simulink model "F16A_Functional"  (R2026a)
settings: Solver=VariableStepAuto
settings Model: DataDictionary=F16A_Functional.sldd  Creator=darsh  LastModifiedBy=darsh

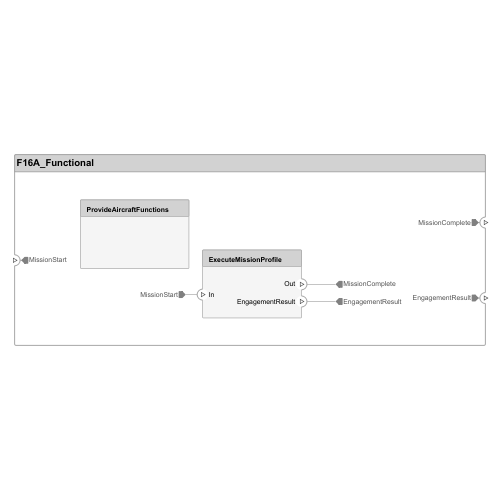
[thumbnail: Simulink's stored preview of the top-level diagram]
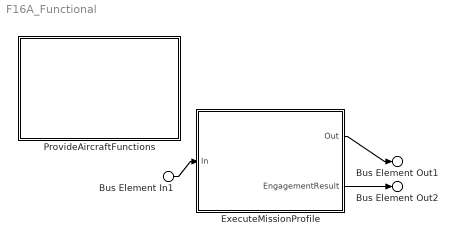
== system F16A_Functional ==
  Bus Element In1 : Inport  PortName=MissionStart
  ExecuteMissionProfile : Subsystem
      settings: PortSchema="{\"entries\":[{\"content\":{\"headerSize\":26,\"margin\":15,\"minimumSpacing\":25,\"sides\":[{\"content\":{\"connectorIds\":[\"In1\"]},\"type\":\"ConnectorPlacement.EquallySpacedRectSide\",\"uuid\":\"f04a52ad-3ae6-4f8c-8d50-829f63627cc8\"},{\"content\":{\"connectorIds\":[\"Out1\",\"Out2\"],\"side\":\"RIGHT\"},\"type\":\"ConnectorPlacement.EquallySpacedRectSide\",\"uuid\":\"fc20b249-404d-406d-9cda-c81cb5f250ae\"},{\"content\":{\"side\":\"TOP\"},\"type\":\"ConnectorPlacement.EquallySpacedRectSide\",\"uuid\":\"dd297750-bae3-47af-9b2d-3c1d29dbfad4\"}]},\"type\":\"ConnectorPlacement.EquallySpacedConnector\",\"uuid\":\"5b4d9ea6-6d9d-4f32-b1f7-36452750b0c8\"}],\"packageUris\":[\"http://schema.mathworks.com/mf0/Connector/R2020b\"],\"version\":\"1.0\"}"
  ProvideAircraftFunctions : Subsystem
      settings: PortSchema="{\"entries\":[{\"content\":{\"headerSize\":26,\"margin\":15,\"minimumSpacing\":25,\"sides\":[{\"content\":{},\"type\":\"ConnectorPlacement.EquallySpacedRectSide\",\"uuid\":\"f04a52ad-3ae6-4f8c-8d50-829f63627cc8\"},{\"content\":{\"side\":\"RIGHT\"},\"type\":\"ConnectorPlacement.EquallySpacedRectSide\",\"uuid\":\"fc20b249-404d-406d-9cda-c81cb5f250ae\"},{\"content\":{\"side\":\"TOP\"},\"type\":\"ConnectorPlacement.EquallySpacedRectSide\",\"uuid\":\"dd297750-bae3-47af-9b2d-3c1d29dbfad4\"}]},\"type\":\"ConnectorPlacement.EquallySpacedConnector\",\"uuid\":\"5b4d9ea6-6d9d-4f32-b1f7-36452750b0c8\"}],\"packageUris\":[\"http://schema.mathworks.com/mf0/Connector/R2020b\"],\"version\":\"1.0\"}"
  Bus Element Out1 : Outport  PortName=MissionComplete
  Bus Element Out2 : Outport  Port=2  PortName=EngagementResult
  wires:
  Bus Element In1/1 -> ExecuteMissionProfile/1(In)
  ExecuteMissionProfile/1(Out) -> Bus Element Out1/1
  ExecuteMissionProfile/2(EngagementResult) -> Bus Element Out2/1

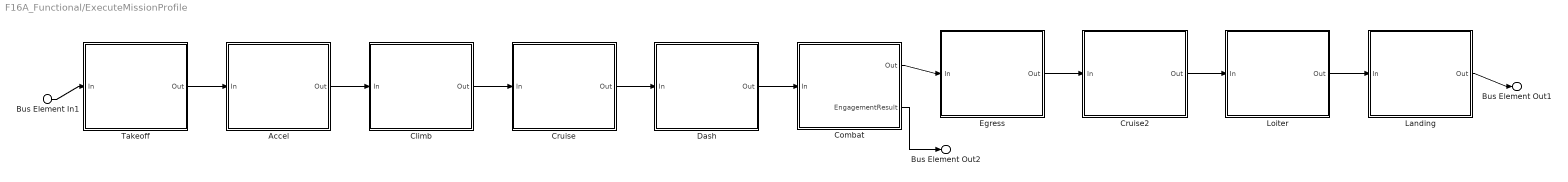
== system F16A_Functional/ExecuteMissionProfile ==
  Bus Element In1 : Inport  PortName=In
  Accel : Subsystem
      settings: PortSchema="{\"entries\":[{\"content\":{\"headerSize\":26,\"margin\":15,\"minimumSpacing\":25,\"sides\":[{\"content\":{\"connectorIds\":[\"In1\"]},\"type\":\"ConnectorPlacement.EquallySpacedRectSide\",\"uuid\":\"f04a52ad-3ae6-4f8c-8d50-829f63627cc8\"},{\"content\":{\"connectorIds\":[\"Out1\"],\"side\":\"RIGHT\"},\"type\":\"ConnectorPlacement.EquallySpacedRectSide\",\"uuid\":\"fc20b249-404d-406d-9cda-c81cb5f250ae\"},{\"content\":{\"side\":\"TOP\"},\"type\":\"ConnectorPlacement.EquallySpacedRectSide\",\"uuid\":\"dd297750-bae3-47af-9b2d-3c1d29dbfad4\"}]},\"type\":\"ConnectorPlacement.EquallySpacedConnector\",\"uuid\":\"5b4d9ea6-6d9d-4f32-b1f7-36452750b0c8\"}],\"packageUris\":[\"http://schema.mathworks.com/mf0/Connector/R2020b\"],\"version\":\"1.0\"}"
  Climb : Subsystem
      settings: PortSchema="{\"entries\":[{\"content\":{\"headerSize\":26,\"margin\":15,\"minimumSpacing\":25,\"sides\":[{\"content\":{\"connectorIds\":[\"In1\"]},\"type\":\"ConnectorPlacement.EquallySpacedRectSide\",\"uuid\":\"f04a52ad-3ae6-4f8c-8d50-829f63627cc8\"},{\"content\":{\"connectorIds\":[\"Out1\"],\"side\":\"RIGHT\"},\"type\":\"ConnectorPlacement.EquallySpacedRectSide\",\"uuid\":\"fc20b249-404d-406d-9cda-c81cb5f250ae\"},{\"content\":{\"side\":\"TOP\"},\"type\":\"ConnectorPlacement.EquallySpacedRectSide\",\"uuid\":\"dd297750-bae3-47af-9b2d-3c1d29dbfad4\"}]},\"type\":\"ConnectorPlacement.EquallySpacedConnector\",\"uuid\":\"5b4d9ea6-6d9d-4f32-b1f7-36452750b0c8\"}],\"packageUris\":[\"http://schema.mathworks.com/mf0/Connector/R2020b\"],\"version\":\"1.0\"}"
  Combat : Subsystem
      settings: PortSchema="{\"entries\":[{\"content\":{\"headerSize\":26,\"margin\":15,\"minimumSpacing\":25,\"sides\":[{\"content\":{\"connectorIds\":[\"In1\"]},\"type\":\"ConnectorPlacement.EquallySpacedRectSide\",\"uuid\":\"f04a52ad-3ae6-4f8c-8d50-829f63627cc8\"},{\"content\":{\"connectorIds\":[\"Out1\",\"Out2\"],\"side\":\"RIGHT\"},\"type\":\"ConnectorPlacement.EquallySpacedRectSide\",\"uuid\":\"fc20b249-404d-406d-9cda-c81cb5f250ae\"},{\"content\":{\"side\":\"TOP\"},\"type\":\"ConnectorPlacement.EquallySpacedRectSide\",\"uuid\":\"dd297750-bae3-47af-9b2d-3c1d29dbfad4\"}]},\"type\":\"ConnectorPlacement.EquallySpacedConnector\",\"uuid\":\"5b4d9ea6-6d9d-4f32-b1f7-36452750b0c8\"}],\"packageUris\":[\"http://schema.mathworks.com/mf0/Connector/R2020b\"],\"version\":\"1.0\"}"
  Cruise : Subsystem
      settings: PortSchema="{\"entries\":[{\"content\":{\"headerSize\":26,\"margin\":15,\"minimumSpacing\":25,\"sides\":[{\"content\":{\"connectorIds\":[\"In1\"]},\"type\":\"ConnectorPlacement.EquallySpacedRectSide\",\"uuid\":\"f04a52ad-3ae6-4f8c-8d50-829f63627cc8\"},{\"content\":{\"connectorIds\":[\"Out1\"],\"side\":\"RIGHT\"},\"type\":\"ConnectorPlacement.EquallySpacedRectSide\",\"uuid\":\"fc20b249-404d-406d-9cda-c81cb5f250ae\"},{\"content\":{\"side\":\"TOP\"},\"type\":\"ConnectorPlacement.EquallySpacedRectSide\",\"uuid\":\"dd297750-bae3-47af-9b2d-3c1d29dbfad4\"}]},\"type\":\"ConnectorPlacement.EquallySpacedConnector\",\"uuid\":\"5b4d9ea6-6d9d-4f32-b1f7-36452750b0c8\"}],\"packageUris\":[\"http://schema.mathworks.com/mf0/Connector/R2020b\"],\"version\":\"1.0\"}"
  Cruise2 : Subsystem
      settings: PortSchema="{\"entries\":[{\"content\":{\"headerSize\":26,\"margin\":15,\"minimumSpacing\":25,\"sides\":[{\"content\":{\"connectorIds\":[\"In1\"]},\"type\":\"ConnectorPlacement.EquallySpacedRectSide\",\"uuid\":\"f04a52ad-3ae6-4f8c-8d50-829f63627cc8\"},{\"content\":{\"connectorIds\":[\"Out1\"],\"side\":\"RIGHT\"},\"type\":\"ConnectorPlacement.EquallySpacedRectSide\",\"uuid\":\"fc20b249-404d-406d-9cda-c81cb5f250ae\"},{\"content\":{\"side\":\"TOP\"},\"type\":\"ConnectorPlacement.EquallySpacedRectSide\",\"uuid\":\"dd297750-bae3-47af-9b2d-3c1d29dbfad4\"}]},\"type\":\"ConnectorPlacement.EquallySpacedConnector\",\"uuid\":\"5b4d9ea6-6d9d-4f32-b1f7-36452750b0c8\"}],\"packageUris\":[\"http://schema.mathworks.com/mf0/Connector/R2020b\"],\"version\":\"1.0\"}"
  Dash : Subsystem
      settings: PortSchema="{\"entries\":[{\"content\":{\"headerSize\":26,\"margin\":15,\"minimumSpacing\":25,\"sides\":[{\"content\":{\"connectorIds\":[\"In1\"]},\"type\":\"ConnectorPlacement.EquallySpacedRectSide\",\"uuid\":\"f04a52ad-3ae6-4f8c-8d50-829f63627cc8\"},{\"content\":{\"connectorIds\":[\"Out1\"],\"side\":\"RIGHT\"},\"type\":\"ConnectorPlacement.EquallySpacedRectSide\",\"uuid\":\"fc20b249-404d-406d-9cda-c81cb5f250ae\"},{\"content\":{\"side\":\"TOP\"},\"type\":\"ConnectorPlacement.EquallySpacedRectSide\",\"uuid\":\"dd297750-bae3-47af-9b2d-3c1d29dbfad4\"}]},\"type\":\"ConnectorPlacement.EquallySpacedConnector\",\"uuid\":\"5b4d9ea6-6d9d-4f32-b1f7-36452750b0c8\"}],\"packageUris\":[\"http://schema.mathworks.com/mf0/Connector/R2020b\"],\"version\":\"1.0\"}"
  Egress : Subsystem
      settings: PortSchema="{\"entries\":[{\"content\":{\"headerSize\":26,\"margin\":15,\"minimumSpacing\":25,\"sides\":[{\"content\":{\"connectorIds\":[\"In1\"]},\"type\":\"ConnectorPlacement.EquallySpacedRectSide\",\"uuid\":\"f04a52ad-3ae6-4f8c-8d50-829f63627cc8\"},{\"content\":{\"connectorIds\":[\"Out1\"],\"side\":\"RIGHT\"},\"type\":\"ConnectorPlacement.EquallySpacedRectSide\",\"uuid\":\"fc20b249-404d-406d-9cda-c81cb5f250ae\"},{\"content\":{\"side\":\"TOP\"},\"type\":\"ConnectorPlacement.EquallySpacedRectSide\",\"uuid\":\"dd297750-bae3-47af-9b2d-3c1d29dbfad4\"}]},\"type\":\"ConnectorPlacement.EquallySpacedConnector\",\"uuid\":\"5b4d9ea6-6d9d-4f32-b1f7-36452750b0c8\"}],\"packageUris\":[\"http://schema.mathworks.com/mf0/Connector/R2020b\"],\"version\":\"1.0\"}"
  Landing : Subsystem
      settings: PortSchema="{\"entries\":[{\"content\":{\"headerSize\":26,\"margin\":15,\"minimumSpacing\":25,\"sides\":[{\"content\":{\"connectorIds\":[\"In1\"]},\"type\":\"ConnectorPlacement.EquallySpacedRectSide\",\"uuid\":\"f04a52ad-3ae6-4f8c-8d50-829f63627cc8\"},{\"content\":{\"connectorIds\":[\"Out1\"],\"side\":\"RIGHT\"},\"type\":\"ConnectorPlacement.EquallySpacedRectSide\",\"uuid\":\"fc20b249-404d-406d-9cda-c81cb5f250ae\"},{\"content\":{\"side\":\"TOP\"},\"type\":\"ConnectorPlacement.EquallySpacedRectSide\",\"uuid\":\"dd297750-bae3-47af-9b2d-3c1d29dbfad4\"}]},\"type\":\"ConnectorPlacement.EquallySpacedConnector\",\"uuid\":\"5b4d9ea6-6d9d-4f32-b1f7-36452750b0c8\"}],\"packageUris\":[\"http://schema.mathworks.com/mf0/Connector/R2020b\"],\"version\":\"1.0\"}"
  Loiter : Subsystem
      settings: PortSchema="{\"entries\":[{\"content\":{\"headerSize\":26,\"margin\":15,\"minimumSpacing\":25,\"sides\":[{\"content\":{\"connectorIds\":[\"In1\"]},\"type\":\"ConnectorPlacement.EquallySpacedRectSide\",\"uuid\":\"f04a52ad-3ae6-4f8c-8d50-829f63627cc8\"},{\"content\":{\"connectorIds\":[\"Out1\"],\"side\":\"RIGHT\"},\"type\":\"ConnectorPlacement.EquallySpacedRectSide\",\"uuid\":\"fc20b249-404d-406d-9cda-c81cb5f250ae\"},{\"content\":{\"side\":\"TOP\"},\"type\":\"ConnectorPlacement.EquallySpacedRectSide\",\"uuid\":\"dd297750-bae3-47af-9b2d-3c1d29dbfad4\"}]},\"type\":\"ConnectorPlacement.EquallySpacedConnector\",\"uuid\":\"5b4d9ea6-6d9d-4f32-b1f7-36452750b0c8\"}],\"packageUris\":[\"http://schema.mathworks.com/mf0/Connector/R2020b\"],\"version\":\"1.0\"}"
  Takeoff : Subsystem
      settings: PortSchema="{\"entries\":[{\"content\":{\"headerSize\":26,\"margin\":15,\"minimumSpacing\":25,\"sides\":[{\"content\":{\"connectorIds\":[\"In1\"]},\"type\":\"ConnectorPlacement.EquallySpacedRectSide\",\"uuid\":\"f04a52ad-3ae6-4f8c-8d50-829f63627cc8\"},{\"content\":{\"connectorIds\":[\"Out1\"],\"side\":\"RIGHT\"},\"type\":\"ConnectorPlacement.EquallySpacedRectSide\",\"uuid\":\"fc20b249-404d-406d-9cda-c81cb5f250ae\"},{\"content\":{\"side\":\"TOP\"},\"type\":\"ConnectorPlacement.EquallySpacedRectSide\",\"uuid\":\"dd297750-bae3-47af-9b2d-3c1d29dbfad4\"}]},\"type\":\"ConnectorPlacement.EquallySpacedConnector\",\"uuid\":\"5b4d9ea6-6d9d-4f32-b1f7-36452750b0c8\"}],\"packageUris\":[\"http://schema.mathworks.com/mf0/Connector/R2020b\"],\"version\":\"1.0\"}"
  Bus Element Out1 : Outport  PortName=Out
  Bus Element Out2 : Outport  Port=2  PortName=EngagementResult
  wires:
  Bus Element In1/1 -> Takeoff/1(In)
  Takeoff/1(Out) -> Accel/1(In)
  Accel/1(Out) -> Climb/1(In)
  Climb/1(Out) -> Cruise/1(In)
  Cruise/1(Out) -> Dash/1(In)
  Combat/2(EngagementResult) -> Bus Element Out2/1
  Dash/1(Out) -> Combat/1(In)
  Combat/1(Out) -> Egress/1(In)
  Cruise2/1(Out) -> Loiter/1(In)
  Egress/1(Out) -> Cruise2/1(In)
  Landing/1(Out) -> Bus Element Out1/1
  Loiter/1(Out) -> Landing/1(In)

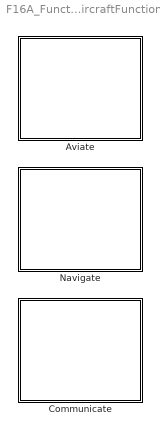
== system F16A_Functional/ProvideAircraftFunctions ==
  Aviate : Subsystem
      settings: PortSchema="{\"entries\":[{\"content\":{\"headerSize\":26,\"margin\":15,\"minimumSpacing\":25,\"sides\":[{\"content\":{},\"type\":\"ConnectorPlacement.EquallySpacedRectSide\",\"uuid\":\"f04a52ad-3ae6-4f8c-8d50-829f63627cc8\"},{\"content\":{\"side\":\"RIGHT\"},\"type\":\"ConnectorPlacement.EquallySpacedRectSide\",\"uuid\":\"fc20b249-404d-406d-9cda-c81cb5f250ae\"},{\"content\":{\"side\":\"TOP\"},\"type\":\"ConnectorPlacement.EquallySpacedRectSide\",\"uuid\":\"dd297750-bae3-47af-9b2d-3c1d29dbfad4\"}]},\"type\":\"ConnectorPlacement.EquallySpacedConnector\",\"uuid\":\"5b4d9ea6-6d9d-4f32-b1f7-36452750b0c8\"}],\"packageUris\":[\"http://schema.mathworks.com/mf0/Connector/R2020b\"],\"version\":\"1.0\"}"
  Communicate : Subsystem
      settings: PortSchema="{\"entries\":[{\"content\":{\"headerSize\":26,\"margin\":15,\"minimumSpacing\":25,\"sides\":[{\"content\":{},\"type\":\"ConnectorPlacement.EquallySpacedRectSide\",\"uuid\":\"f04a52ad-3ae6-4f8c-8d50-829f63627cc8\"},{\"content\":{\"side\":\"RIGHT\"},\"type\":\"ConnectorPlacement.EquallySpacedRectSide\",\"uuid\":\"fc20b249-404d-406d-9cda-c81cb5f250ae\"},{\"content\":{\"side\":\"TOP\"},\"type\":\"ConnectorPlacement.EquallySpacedRectSide\",\"uuid\":\"dd297750-bae3-47af-9b2d-3c1d29dbfad4\"}]},\"type\":\"ConnectorPlacement.EquallySpacedConnector\",\"uuid\":\"5b4d9ea6-6d9d-4f32-b1f7-36452750b0c8\"}],\"packageUris\":[\"http://schema.mathworks.com/mf0/Connector/R2020b\"],\"version\":\"1.0\"}"
  Navigate : Subsystem
      settings: PortSchema="{\"entries\":[{\"content\":{\"headerSize\":26,\"margin\":15,\"minimumSpacing\":25,\"sides\":[{\"content\":{},\"type\":\"ConnectorPlacement.EquallySpacedRectSide\",\"uuid\":\"f04a52ad-3ae6-4f8c-8d50-829f63627cc8\"},{\"content\":{\"side\":\"RIGHT\"},\"type\":\"ConnectorPlacement.EquallySpacedRectSide\",\"uuid\":\"fc20b249-404d-406d-9cda-c81cb5f250ae\"},{\"content\":{\"side\":\"TOP\"},\"type\":\"ConnectorPlacement.EquallySpacedRectSide\",\"uuid\":\"dd297750-bae3-47af-9b2d-3c1d29dbfad4\"}]},\"type\":\"ConnectorPlacement.EquallySpacedConnector\",\"uuid\":\"5b4d9ea6-6d9d-4f32-b1f7-36452750b0c8\"}],\"packageUris\":[\"http://schema.mathworks.com/mf0/Connector/R2020b\"],\"version\":\"1.0\"}"

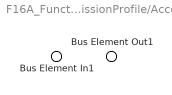
== system F16A_Functional/ExecuteMissionProfile/Accel ==
  Bus Element In1 : Inport  PortName=In
  Bus Element Out1 : Outport  PortName=Out

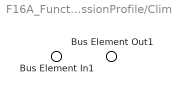
== system F16A_Functional/ExecuteMissionProfile/Climb ==
  Bus Element In1 : Inport  PortName=In
  Bus Element Out1 : Outport  PortName=Out

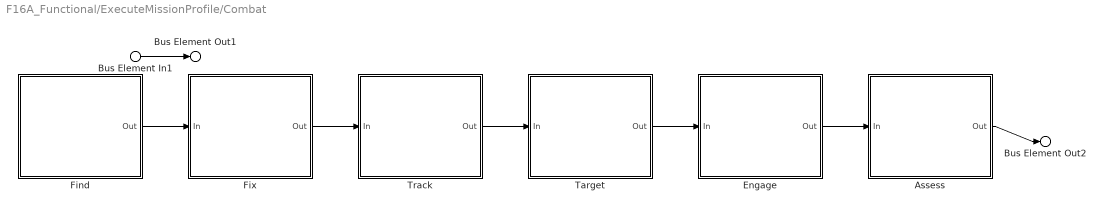
== system F16A_Functional/ExecuteMissionProfile/Combat ==
  Bus Element In1 : Inport  PortName=In
  Assess : Subsystem
      settings: PortSchema="{\"entries\":[{\"content\":{\"headerSize\":26,\"margin\":15,\"minimumSpacing\":25,\"sides\":[{\"content\":{\"connectorIds\":[\"In1\"]},\"type\":\"ConnectorPlacement.EquallySpacedRectSide\",\"uuid\":\"f04a52ad-3ae6-4f8c-8d50-829f63627cc8\"},{\"content\":{\"connectorIds\":[\"Out1\"],\"side\":\"RIGHT\"},\"type\":\"ConnectorPlacement.EquallySpacedRectSide\",\"uuid\":\"fc20b249-404d-406d-9cda-c81cb5f250ae\"},{\"content\":{\"side\":\"TOP\"},\"type\":\"ConnectorPlacement.EquallySpacedRectSide\",\"uuid\":\"dd297750-bae3-47af-9b2d-3c1d29dbfad4\"}]},\"type\":\"ConnectorPlacement.EquallySpacedConnector\",\"uuid\":\"5b4d9ea6-6d9d-4f32-b1f7-36452750b0c8\"}],\"packageUris\":[\"http://schema.mathworks.com/mf0/Connector/R2020b\"],\"version\":\"1.0\"}"
  Engage : Subsystem
      settings: PortSchema="{\"entries\":[{\"content\":{\"headerSize\":26,\"margin\":15,\"minimumSpacing\":25,\"sides\":[{\"content\":{\"connectorIds\":[\"In1\"]},\"type\":\"ConnectorPlacement.EquallySpacedRectSide\",\"uuid\":\"f04a52ad-3ae6-4f8c-8d50-829f63627cc8\"},{\"content\":{\"connectorIds\":[\"Out1\"],\"side\":\"RIGHT\"},\"type\":\"ConnectorPlacement.EquallySpacedRectSide\",\"uuid\":\"fc20b249-404d-406d-9cda-c81cb5f250ae\"},{\"content\":{\"side\":\"TOP\"},\"type\":\"ConnectorPlacement.EquallySpacedRectSide\",\"uuid\":\"dd297750-bae3-47af-9b2d-3c1d29dbfad4\"}]},\"type\":\"ConnectorPlacement.EquallySpacedConnector\",\"uuid\":\"5b4d9ea6-6d9d-4f32-b1f7-36452750b0c8\"}],\"packageUris\":[\"http://schema.mathworks.com/mf0/Connector/R2020b\"],\"version\":\"1.0\"}"
  Find : Subsystem
      settings: PortSchema="{\"entries\":[{\"content\":{\"headerSize\":26,\"margin\":15,\"minimumSpacing\":25,\"sides\":[{\"content\":{},\"type\":\"ConnectorPlacement.EquallySpacedRectSide\",\"uuid\":\"f04a52ad-3ae6-4f8c-8d50-829f63627cc8\"},{\"content\":{\"connectorIds\":[\"Out1\"],\"side\":\"RIGHT\"},\"type\":\"ConnectorPlacement.EquallySpacedRectSide\",\"uuid\":\"fc20b249-404d-406d-9cda-c81cb5f250ae\"},{\"content\":{\"side\":\"TOP\"},\"type\":\"ConnectorPlacement.EquallySpacedRectSide\",\"uuid\":\"dd297750-bae3-47af-9b2d-3c1d29dbfad4\"}]},\"type\":\"ConnectorPlacement.EquallySpacedConnector\",\"uuid\":\"5b4d9ea6-6d9d-4f32-b1f7-36452750b0c8\"}],\"packageUris\":[\"http://schema.mathworks.com/mf0/Connector/R2020b\"],\"version\":\"1.0\"}"
  Fix : Subsystem
      settings: PortSchema="{\"entries\":[{\"content\":{\"headerSize\":26,\"margin\":15,\"minimumSpacing\":25,\"sides\":[{\"content\":{\"connectorIds\":[\"In1\"]},\"type\":\"ConnectorPlacement.EquallySpacedRectSide\",\"uuid\":\"f04a52ad-3ae6-4f8c-8d50-829f63627cc8\"},{\"content\":{\"connectorIds\":[\"Out1\"],\"side\":\"RIGHT\"},\"type\":\"ConnectorPlacement.EquallySpacedRectSide\",\"uuid\":\"fc20b249-404d-406d-9cda-c81cb5f250ae\"},{\"content\":{\"side\":\"TOP\"},\"type\":\"ConnectorPlacement.EquallySpacedRectSide\",\"uuid\":\"dd297750-bae3-47af-9b2d-3c1d29dbfad4\"}]},\"type\":\"ConnectorPlacement.EquallySpacedConnector\",\"uuid\":\"5b4d9ea6-6d9d-4f32-b1f7-36452750b0c8\"}],\"packageUris\":[\"http://schema.mathworks.com/mf0/Connector/R2020b\"],\"version\":\"1.0\"}"
  Target : Subsystem
      settings: PortSchema="{\"entries\":[{\"content\":{\"headerSize\":26,\"margin\":15,\"minimumSpacing\":25,\"sides\":[{\"content\":{\"connectorIds\":[\"In1\"]},\"type\":\"ConnectorPlacement.EquallySpacedRectSide\",\"uuid\":\"f04a52ad-3ae6-4f8c-8d50-829f63627cc8\"},{\"content\":{\"connectorIds\":[\"Out1\"],\"side\":\"RIGHT\"},\"type\":\"ConnectorPlacement.EquallySpacedRectSide\",\"uuid\":\"fc20b249-404d-406d-9cda-c81cb5f250ae\"},{\"content\":{\"side\":\"TOP\"},\"type\":\"ConnectorPlacement.EquallySpacedRectSide\",\"uuid\":\"dd297750-bae3-47af-9b2d-3c1d29dbfad4\"}]},\"type\":\"ConnectorPlacement.EquallySpacedConnector\",\"uuid\":\"5b4d9ea6-6d9d-4f32-b1f7-36452750b0c8\"}],\"packageUris\":[\"http://schema.mathworks.com/mf0/Connector/R2020b\"],\"version\":\"1.0\"}"
  Track : Subsystem
      settings: PortSchema="{\"entries\":[{\"content\":{\"headerSize\":26,\"margin\":15,\"minimumSpacing\":25,\"sides\":[{\"content\":{\"connectorIds\":[\"In1\"]},\"type\":\"ConnectorPlacement.EquallySpacedRectSide\",\"uuid\":\"f04a52ad-3ae6-4f8c-8d50-829f63627cc8\"},{\"content\":{\"connectorIds\":[\"Out1\"],\"side\":\"RIGHT\"},\"type\":\"ConnectorPlacement.EquallySpacedRectSide\",\"uuid\":\"fc20b249-404d-406d-9cda-c81cb5f250ae\"},{\"content\":{\"side\":\"TOP\"},\"type\":\"ConnectorPlacement.EquallySpacedRectSide\",\"uuid\":\"dd297750-bae3-47af-9b2d-3c1d29dbfad4\"}]},\"type\":\"ConnectorPlacement.EquallySpacedConnector\",\"uuid\":\"5b4d9ea6-6d9d-4f32-b1f7-36452750b0c8\"}],\"packageUris\":[\"http://schema.mathworks.com/mf0/Connector/R2020b\"],\"version\":\"1.0\"}"
  Bus Element Out1 : Outport  PortName=Out
  Bus Element Out2 : Outport  Port=2  PortName=EngagementResult
  wires:
  Bus Element In1/1 -> Bus Element Out1/1
  Fix/1(Out) -> Track/1(In)
  Find/1(Out) -> Fix/1(In)
  Target/1(Out) -> Engage/1(In)
  Track/1(Out) -> Target/1(In)
  Assess/1(Out) -> Bus Element Out2/1
  Engage/1(Out) -> Assess/1(In)

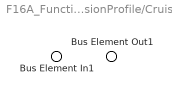
== system F16A_Functional/ExecuteMissionProfile/Cruise ==
  Bus Element In1 : Inport  PortName=In
  Bus Element Out1 : Outport  PortName=Out

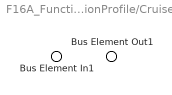
== system F16A_Functional/ExecuteMissionProfile/Cruise2 ==
  Bus Element In1 : Inport  PortName=In
  Bus Element Out1 : Outport  PortName=Out

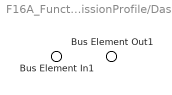
== system F16A_Functional/ExecuteMissionProfile/Dash ==
  Bus Element In1 : Inport  PortName=In
  Bus Element Out1 : Outport  PortName=Out

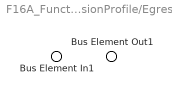
== system F16A_Functional/ExecuteMissionProfile/Egress ==
  Bus Element In1 : Inport  PortName=In
  Bus Element Out1 : Outport  PortName=Out

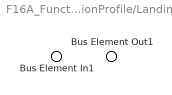
== system F16A_Functional/ExecuteMissionProfile/Landing ==
  Bus Element In1 : Inport  PortName=In
  Bus Element Out1 : Outport  PortName=Out

== system F16A_Functional/ExecuteMissionProfile/Loiter ==
  Bus Element In1 : Inport  PortName=In
  Bus Element Out1 : Outport  PortName=Out

== system F16A_Functional/ExecuteMissionProfile/Takeoff ==
  Bus Element In1 : Inport  PortName=In
  Bus Element Out1 : Outport  PortName=Out

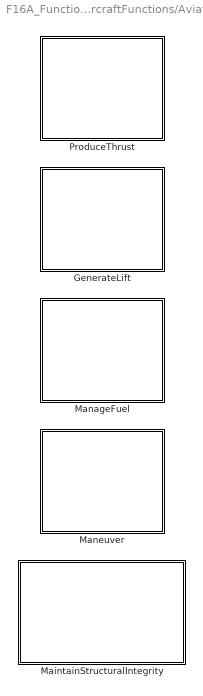
== system F16A_Functional/ProvideAircraftFunctions/Aviate ==
  GenerateLift : Subsystem
      settings: PortSchema="{\"entries\":[{\"content\":{\"headerSize\":26,\"margin\":15,\"minimumSpacing\":25,\"sides\":[{\"content\":{},\"type\":\"ConnectorPlacement.EquallySpacedRectSide\",\"uuid\":\"f04a52ad-3ae6-4f8c-8d50-829f63627cc8\"},{\"content\":{\"side\":\"RIGHT\"},\"type\":\"ConnectorPlacement.EquallySpacedRectSide\",\"uuid\":\"fc20b249-404d-406d-9cda-c81cb5f250ae\"},{\"content\":{\"side\":\"TOP\"},\"type\":\"ConnectorPlacement.EquallySpacedRectSide\",\"uuid\":\"dd297750-bae3-47af-9b2d-3c1d29dbfad4\"}]},\"type\":\"ConnectorPlacement.EquallySpacedConnector\",\"uuid\":\"5b4d9ea6-6d9d-4f32-b1f7-36452750b0c8\"}],\"packageUris\":[\"http://schema.mathworks.com/mf0/Connector/R2020b\"],\"version\":\"1.0\"}"
  MaintainStructuralIntegrity : Subsystem
      settings: PortSchema="{\"entries\":[{\"content\":{\"headerSize\":26,\"margin\":15,\"minimumSpacing\":25,\"sides\":[{\"content\":{},\"type\":\"ConnectorPlacement.EquallySpacedRectSide\",\"uuid\":\"f04a52ad-3ae6-4f8c-8d50-829f63627cc8\"},{\"content\":{\"side\":\"RIGHT\"},\"type\":\"ConnectorPlacement.EquallySpacedRectSide\",\"uuid\":\"fc20b249-404d-406d-9cda-c81cb5f250ae\"},{\"content\":{\"side\":\"TOP\"},\"type\":\"ConnectorPlacement.EquallySpacedRectSide\",\"uuid\":\"dd297750-bae3-47af-9b2d-3c1d29dbfad4\"}]},\"type\":\"ConnectorPlacement.EquallySpacedConnector\",\"uuid\":\"5b4d9ea6-6d9d-4f32-b1f7-36452750b0c8\"}],\"packageUris\":[\"http://schema.mathworks.com/mf0/Connector/R2020b\"],\"version\":\"1.0\"}"
  ManageFuel : Subsystem
      settings: PortSchema="{\"entries\":[{\"content\":{\"headerSize\":26,\"margin\":15,\"minimumSpacing\":25,\"sides\":[{\"content\":{},\"type\":\"ConnectorPlacement.EquallySpacedRectSide\",\"uuid\":\"f04a52ad-3ae6-4f8c-8d50-829f63627cc8\"},{\"content\":{\"side\":\"RIGHT\"},\"type\":\"ConnectorPlacement.EquallySpacedRectSide\",\"uuid\":\"fc20b249-404d-406d-9cda-c81cb5f250ae\"},{\"content\":{\"side\":\"TOP\"},\"type\":\"ConnectorPlacement.EquallySpacedRectSide\",\"uuid\":\"dd297750-bae3-47af-9b2d-3c1d29dbfad4\"}]},\"type\":\"ConnectorPlacement.EquallySpacedConnector\",\"uuid\":\"5b4d9ea6-6d9d-4f32-b1f7-36452750b0c8\"}],\"packageUris\":[\"http://schema.mathworks.com/mf0/Connector/R2020b\"],\"version\":\"1.0\"}"
  Maneuver : Subsystem
      settings: PortSchema="{\"entries\":[{\"content\":{\"headerSize\":26,\"margin\":15,\"minimumSpacing\":25,\"sides\":[{\"content\":{},\"type\":\"ConnectorPlacement.EquallySpacedRectSide\",\"uuid\":\"f04a52ad-3ae6-4f8c-8d50-829f63627cc8\"},{\"content\":{\"side\":\"RIGHT\"},\"type\":\"ConnectorPlacement.EquallySpacedRectSide\",\"uuid\":\"fc20b249-404d-406d-9cda-c81cb5f250ae\"},{\"content\":{\"side\":\"TOP\"},\"type\":\"ConnectorPlacement.EquallySpacedRectSide\",\"uuid\":\"dd297750-bae3-47af-9b2d-3c1d29dbfad4\"}]},\"type\":\"ConnectorPlacement.EquallySpacedConnector\",\"uuid\":\"5b4d9ea6-6d9d-4f32-b1f7-36452750b0c8\"}],\"packageUris\":[\"http://schema.mathworks.com/mf0/Connector/R2020b\"],\"version\":\"1.0\"}"
  ProduceThrust : Subsystem
      settings: PortSchema="{\"entries\":[{\"content\":{\"headerSize\":26,\"margin\":15,\"minimumSpacing\":25,\"sides\":[{\"content\":{},\"type\":\"ConnectorPlacement.EquallySpacedRectSide\",\"uuid\":\"f04a52ad-3ae6-4f8c-8d50-829f63627cc8\"},{\"content\":{\"side\":\"RIGHT\"},\"type\":\"ConnectorPlacement.EquallySpacedRectSide\",\"uuid\":\"fc20b249-404d-406d-9cda-c81cb5f250ae\"},{\"content\":{\"side\":\"TOP\"},\"type\":\"ConnectorPlacement.EquallySpacedRectSide\",\"uuid\":\"dd297750-bae3-47af-9b2d-3c1d29dbfad4\"}]},\"type\":\"ConnectorPlacement.EquallySpacedConnector\",\"uuid\":\"5b4d9ea6-6d9d-4f32-b1f7-36452750b0c8\"}],\"packageUris\":[\"http://schema.mathworks.com/mf0/Connector/R2020b\"],\"version\":\"1.0\"}"

== system F16A_Functional/ProvideAircraftFunctions/Communicate ==

== system F16A_Functional/ProvideAircraftFunctions/Navigate ==

== system F16A_Functional/ExecuteMissionProfile/Combat/Assess ==
  Bus Element In1 : Inport  PortName=In
  Bus Element Out1 : Outport  PortName=Out

== system F16A_Functional/ExecuteMissionProfile/Combat/Engage ==
  Bus Element In1 : Inport  PortName=In
  Bus Element Out1 : Outport  PortName=Out

== system F16A_Functional/ExecuteMissionProfile/Combat/Find ==
  Bus Element Out1 : Outport  PortName=Out

== system F16A_Functional/ExecuteMissionProfile/Combat/Fix ==
  Bus Element In1 : Inport  PortName=In
  Bus Element Out1 : Outport  PortName=Out

== system F16A_Functional/ExecuteMissionProfile/Combat/Target ==
  Bus Element In1 : Inport  PortName=In
  Bus Element Out1 : Outport  PortName=Out

== system F16A_Functional/ExecuteMissionProfile/Combat/Track ==
  Bus Element In1 : Inport  PortName=In
  Bus Element Out1 : Outport  PortName=Out

== system F16A_Functional/ProvideAircraftFunctions/Aviate/GenerateLift ==

== system F16A_Functional/ProvideAircraftFunctions/Aviate/MaintainStructuralIntegrity ==

== system F16A_Functional/ProvideAircraftFunctions/Aviate/ManageFuel ==

== system F16A_Functional/ProvideAircraftFunctions/Aviate/Maneuver ==

== system F16A_Functional/ProvideAircraftFunctions/Aviate/ProduceThrust ==
